simulink subsystem "Mk2NeckWrapper"  (R2025a)
settings: Solver=VariableStepAuto  StartTime=0.0  StopTime=10.0  RelTol=1e-3
undefined symbols (not defined in the file): Joint1_B, Joint1_F, Joint2_B, Joint2_F, Joint3_B, Joint3_F, Motor1, Motor2, Payload_base_frame, Transmission1_Stage1, Transmission1_Stage2, Transmission2_Stage1, Transmission2_Stage2, Transmission3_Stage1, X, Y, Z
libraries: sm_lib x1
settings Model: DataDictionary=neck_mk3.sldd  EnableAccessToBaseWorkspace=off  Creator=upattacini  LastModifiedBy=upattacini
settings RTWCC: GPUComputeCapability=3.5

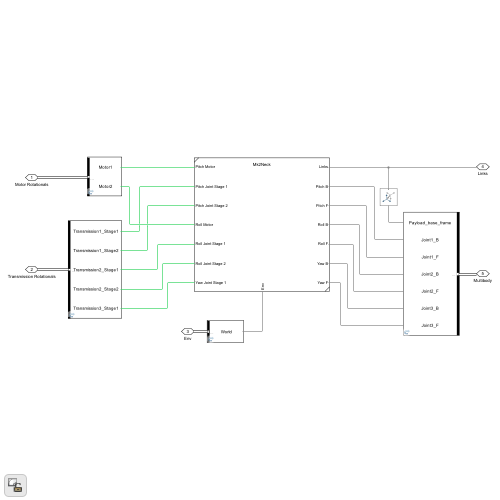
[thumbnail: Simulink's stored preview of the top-level diagram]
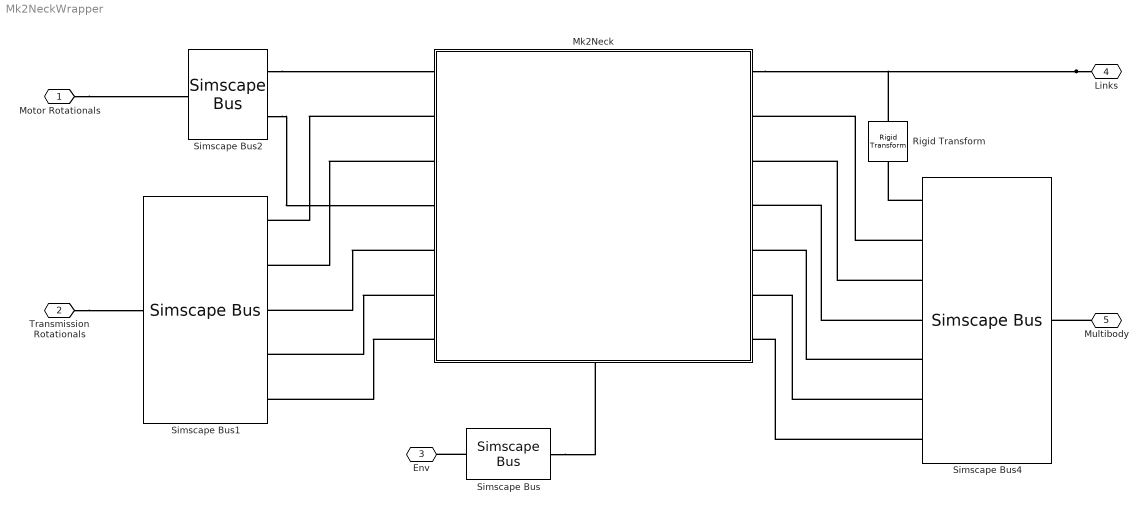
== system Mk2NeckWrapper ==
  Mk2Neck : Subsystem  ReferencedSubsystem=Mk2Neck
      settings: PermitHierarchicalResolution=None  PortSchema="{\"entries\":[{\"content\":{\"sides\":[{\"content\":{\"connectorIds\":[\"LConn1\",\"LConn2\",\"LConn3\",\"LConn4\",\"LConn5\",\"LConn6\",\"LConn7\"]},\"type\":\"ConnectorPlacement.EquallySpacedRectSide\",\"uuid\":\"5b2764b2-b856-4686-b351-9b266f955fd8\"},{\"content\":{\"connectorIds\":[\"RConn1\",\"RConn3\",\"RConn4\",\"RConn5\",\"RConn6\",\"RConn7\",\"RConn8\"],\"side\":\"RIGHT\"},\"type\":\"ConnectorPlacement.EquallySpacedRectSide\",\"uuid\":\"d0e082f1-429c-4ec8-8d3c-28dcb5a8bf62\"},{\"content\":{\"side\":\"TOP\"},\"type\":\"ConnectorPlacement.EquallySpacedRectSide\",\"uuid\":\"4ede2f6a-8a03-4dea-aacb-7b97af4e79a7\"},{\"content\":{\"connectorIds\":[\"RConn2\"],\"side\":\"BOTTOM\"},\"type\":\"ConnectorPlacement.EquallySpacedRectSide\",\"uuid\":\"965e68a2-8eb6-4733-a0cf-8fe75774ceed\"}]},\"type\":\"ConnectorPlacement.EquallySpacedConnector\",\"uuid\":\"b45bb07b-977f-4590-ab88-951f4e9eebf0\"}],\"packageUris\":[\"http://schema.mathworks.com/mf0/Connector/R2020b\"],\"version\":\"1.0\"}"
  Rigid Transform : sm_lib/Frames and Transforms/Rigid Transform  RotationMethod=RotationMatrix  FollAlignAxisA=+X  BaseAlignAxisA=+Y  FollAlignAxisB=+Y  BaseAlignAxisB=+Z  RotationStandardAxis=+Y  RotationAngle=-90  RotationAngleUnits=deg  RotationArbitraryAxis=[0 0 1]  RotationSequenceAxes=FollowerAxes  RotationSequence=XYX  RotationSequenceAngles=[0 0 0]  RotationSequenceAnglesUnits=deg  RotationMatrix=[0 1 0; 0 0 1; 1 0 0]  Quaternion=[1 0 0 0]  TranslationMethod=None  TranslationCartesianOffset=[0 0 0]  TranslationCartesianOffsetUnits=m  TranslationStandardAxis=+Z  TranslationStandardOffset=0  TranslationStandardOffsetUnits=m  TranslationROffset=0  TranslationROffsetUnits=m  TranslationThetaOffset=0  TranslationThetaOffsetUnits=deg  TranslationZOffset=0  TranslationZOffsetUnits=m
  Simscape Bus : SimscapeBus  HierarchyStrings=World  ConnectionType=Bus: Physical_Environment
  Simscape Bus1 : SimscapeBus  HierarchyStrings=Transmission1_Stage1;Transmission1_Stage2;Transmission2_Stage1;Transmission2_Stage2;Transmission3_Stage1  ConnectionType=Bus: Physical_TransmissionRotationals
  Simscape Bus2 : SimscapeBus  HierarchyStrings=Motor1;Motor2  ConnectionType=Bus: Physical_MotorRotationals
  Simscape Bus4 : SimscapeBus  HierarchyStrings=Payload_base_frame;Joint1_B;Joint1_F;Joint2_B;Joint2_F;Joint3_B;Joint3_F  ConnectionType=Bus: Physical_Multibody
  Motor Rotationals : PMIOPort  Side=Left
  Transmission Rotationals : PMIOPort  Port=2  Side=Left
  Env : PMIOPort  Port=3  Side=Right
  Links : PMIOPort  Port=4  Side=Right
  Multibody : PMIOPort  Port=5  Side=Right
  connections:
  Links/RConn1 -- Rigid Transform/LConn1 -- Mk2Neck/RConn1
  Simscape Bus/RConn1 -- Env/RConn1
  Motor Rotationals/RConn1 -- Simscape Bus2/RConn1
  Simscape Bus/LConn1 -- Mk2Neck/RConn2
  Simscape Bus2/LConn1 -- Mk2Neck/LConn1
  Simscape Bus2/LConn2 -- Mk2Neck/LConn4
  Mk2Neck/LConn2 -- Simscape Bus1/LConn1
  Mk2Neck/LConn3 -- Simscape Bus1/LConn2
  Mk2Neck/LConn5 -- Simscape Bus1/LConn3
  Mk2Neck/LConn6 -- Simscape Bus1/LConn4
  Mk2Neck/LConn7 -- Simscape Bus1/LConn5
  Transmission Rotationals/RConn1 -- Simscape Bus1/RConn1
  Multibody/RConn1 -- Simscape Bus4/RConn1
  Simscape Bus4/LConn2 -- Mk2Neck/RConn3
  Simscape Bus4/LConn3 -- Mk2Neck/RConn4
  Simscape Bus4/LConn4 -- Mk2Neck/RConn5
  Simscape Bus4/LConn5 -- Mk2Neck/RConn6
  Simscape Bus4/LConn6 -- Mk2Neck/RConn7
  Simscape Bus4/LConn7 -- Mk2Neck/RConn8
  Simscape Bus4/LConn1 -- Rigid Transform/RConn1
